simulink model "AFDNFSmodelSPA"  (Simulink 9.0)
settings: Solver=ode45  StartTime=0.0  StopTime=100  FixedStep=1e-3  RelTol=1e-6  EnableMultiTasking=on
InitFcn:
  | run('Methods/AFDSimInit')
values from neighbouring files (symbols this model uses):
  nfs = TransferFunction('Plot','true')    [Main.m]    (also in NFSDatabase.sldd = SI
                Imperial
                28184.4409185639)
undefined symbols (not defined in the file or in its folder): desired, F, K_lat, K_long, Kobsvlat, Kobsvlong, lat, latsys, Light, long, longsys, MIL, Newton, Raphson, sigbuilder_block
libraries: aerolibwind2 x2, sharedutil x1
(part 2 of 3)

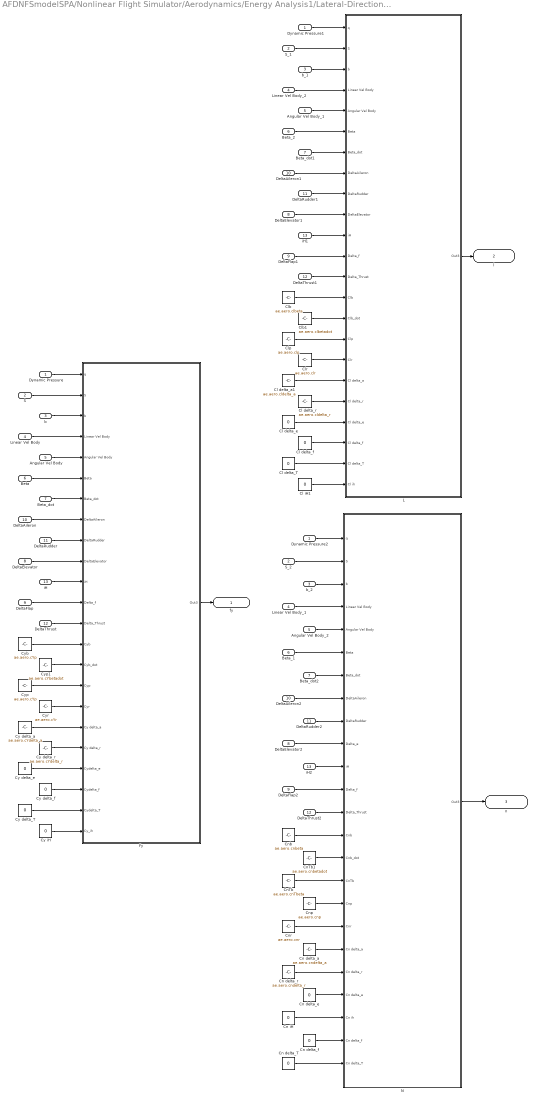
== system AFDNFSmodelSPA/Nonlinear Flight Simulator/Aerodynamics/Energy Analysis1/Lateral-Directional1 ==
  Dynamic Pressure : Inport
  S : Inport  Port=2
  b : Inport  Port=3
  Linear Vel Body : Inport  Port=4
  Angular Vel Body : Inport  Port=5
  Beta : Inport  Port=6
  Beta_dot : Inport  Port=7
  DeltaElevator : Inport  Port=8
  DeltaFlap : Inport  Port=9
  DeltaAileron : Inport  Port=10
  DeltaRudder : Inport  Port=11
  DeltaThrust : Inport  Port=12
  iH : Inport  Port=13
  Angular Vel Body_1 : InportShadow  Port=5
  Angular Vel Body_2 : InportShadow  Port=5
  Beta_1 : InportShadow  Port=6
  Beta_2 : InportShadow  Port=6
  Beta_dot1 : InportShadow  Port=7
  Beta_dot2 : InportShadow  Port=7
  Cl delta_T : Constant  Value=0
  Cl delta_a1 : Constant  Value=ae.aero.cldelta_a
  Cl delta_e : Constant  Value=0
  Cl delta_f : Constant  Value=0
  Cl delta_r : Constant  Value=ae.aero.cldelta_r
  Cl iH1 : Constant  Value=0
  Clb : Constant  Value=ae.aero.clbeta
  Clb1 : Constant  Value=ae.aero.clbetadot
  Clp : Constant  Value=ae.aero.clp
  Clr : Constant  Value=ae.aero.clr
  Cn delta_T : Constant  Value=0
  Cn delta_a : Constant  Value=ae.aero.cndelta_a
  Cn delta_e : Constant  Value=0
  Cn delta_f : Constant  Value=0
  Cn delta_r : Constant  Value=ae.aero.cndelta_r
  Cn iH : Constant  Value=0
  CnTb : Constant  Value=ae.aero.cnTbeta
  CnTb1 : Constant  Value=ae.aero.cnbetadot
  Cnb : Constant  Value=ae.aero.cnbeta
  Cnp : Constant  Value=ae.aero.cnp
  Cnr : Constant  Value=ae.aero.cnr
  Cy delta_T : Constant  Value=0
  Cy delta_a : Constant  Value=ae.aero.cYdelta_a
  Cy delta_e : Constant  Value=0
  Cy delta_f : Constant  Value=0
  Cy delta_r : Constant  Value=ae.aero.cYdelta_r
  Cy iH : Constant  Value=0
  Cyb : Constant  Value=ae.aero.cYp
  Cyp : Constant  Value=ae.aero.cYp
  Cyp1 : Constant  Value=ae.aero.cYbetadot
  Cyr : Constant  Value=ae.aero.cYr
  DeltaAileron1 : InportShadow  Port=10
  DeltaAileron2 : InportShadow  Port=10
  DeltaElevator1 : InportShadow  Port=8
  DeltaElevator2 : InportShadow  Port=8
  DeltaFlap1 : InportShadow  Port=9
  DeltaFlap2 : InportShadow  Port=9
  DeltaRudder1 : InportShadow  Port=11
  DeltaRudder2 : InportShadow  Port=11
  DeltaThrust1 : InportShadow  Port=12
  DeltaThrust2 : InportShadow  Port=12
  Dynamic Pressure1 : InportShadow
  Dynamic Pressure2 : InportShadow
  Fy : Subsystem
  L : Subsystem
  Linear Vel Body_1 : InportShadow  Port=4
  Linear Vel Body_2 : InportShadow  Port=4
  N : Subsystem
  S_1 : InportShadow  Port=2
  S_2 : InportShadow  Port=2
  b_1 : InportShadow  Port=3
  b_2 : InportShadow  Port=3
  iH1 : InportShadow  Port=13
  iH2 : InportShadow  Port=13
  fy : Outport
  l : Outport  Port=2
  n : Outport  Port=3
  wires:
  L/1(Out3) -> l/1
  N/1(Out3) -> n/1
  Fy/1(Out3) -> fy/1
  Dynamic Pressure/1 -> Fy/1(q)
  S/1 -> Fy/2(S)
  b/1 -> Fy/3(b)
  Linear Vel Body/1 -> Fy/4(Linear Vel Body)
  Angular Vel Body/1 -> Fy/5(Angular Vel Body)
  Beta/1 -> Fy/6(Beta)
  Beta_dot/1 -> Fy/7(Beta_dot)
  DeltaAileron/1 -> Fy/8(DeltaAileron)
  DeltaRudder/1 -> Fy/9(DeltaRudder)
  iH/1 -> Fy/11(iH)
  DeltaElevator/1 -> Fy/10(DeltaElevator)
  DeltaFlap/1 -> Fy/12(Delta_f)
  DeltaThrust/1 -> Fy/13(Delta_Thrust)
  DeltaRudder2/1 -> N/9(DeltaRudder)
  DeltaAileron2/1 -> N/8(DeltaAileron)
  Dynamic Pressure2/1 -> N/1(q)
  DeltaThrust2/1 -> N/13(Delta_Thrust)
  b_2/1 -> N/3(b)
  Angular Vel Body_2/1 -> N/5(Angular Vel Body)
  Linear Vel Body_1/1 -> N/4(Linear Vel Body)
  iH2/1 -> N/11(iH)
  Beta_dot2/1 -> N/7(Beta_dot)
  S_2/1 -> N/2(S)
  DeltaElevator2/1 -> N/10(Delta_e)
  DeltaFlap2/1 -> N/12(Delta_f)
  Beta_1/1 -> N/6(Beta)
  Cyb/1 -> Fy/14(Cyb)
  Cyp/1 -> Fy/16(Cyp)
  Cyr/1 -> Fy/17(Cyr)
  Cy delta_a/1 -> Fy/18(Cy delta_a)
  Cy delta_r/1 -> Fy/19(Cy delta_r)
  Cy delta_e/1 -> Fy/20(Cydelta_e)
  Cy delta_f/1 -> Fy/21(Cydelta_f)
  Cy delta_T/1 -> Fy/22(Cydelta_T)
  Cy iH/1 -> Fy/23(Cy_ih)
  Cnb/1 -> N/14(Cnb)
  Cnp/1 -> N/17(Cnp)
  Cn delta_T/1 -> N/24(Cn delta_T)
  CnTb/1 -> N/16(CnTb)
  Cn delta_a/1 -> N/19(Cn delta_a)
  Cn delta_e/1 -> N/21(Cn delta_e)
  Cn delta_r/1 -> N/20(Cn delta_r)
  Cn iH/1 -> N/22(Cn ih)
  Cn delta_f/1 -> N/23(Cn delta_f)
  Cnr/1 -> N/18(Cnr)
  Clb/1 -> L/14(Clb)
  Clp/1 -> L/16(Clp)
  Cl delta_a1/1 -> L/18(Cl delta_a)
  b_1/1 -> L/3(b)
  Dynamic Pressure1/1 -> L/1(q)
  Angular Vel Body_1/1 -> L/5(Angular Vel Body)
  iH1/1 -> L/11(iH)
  DeltaRudder1/1 -> L/9(DeltaRudder)
  DeltaThrust1/1 -> L/13(Delta_Thrust)
  Beta_dot1/1 -> L/7(Beta_dot)
  Beta_2/1 -> L/6(Beta)
  DeltaAileron1/1 -> L/8(DeltaAileron)
  DeltaFlap1/1 -> L/12(Delta_f)
  DeltaElevator1/1 -> L/10(DeltaElevator)
  Linear Vel Body_2/1 -> L/4(Linear Vel Body)
  S_1/1 -> L/2(S)
  Clr/1 -> L/17(Clr)
  Cl delta_e/1 -> L/20(Cl delta_e)
  Cl delta_T/1 -> L/22(Cl delta_T)
  Cl delta_f/1 -> L/21(Cl delta_f)
  Cl delta_r/1 -> L/19(Cl delta_r)
  Cl iH1/1 -> L/23(Cl ih)
  Clb1/1 -> L/15(Clb_dot)
  CnTb1/1 -> N/15(Cnb_dot)
  Cyp1/1 -> Fy/15(Cyb_dot)

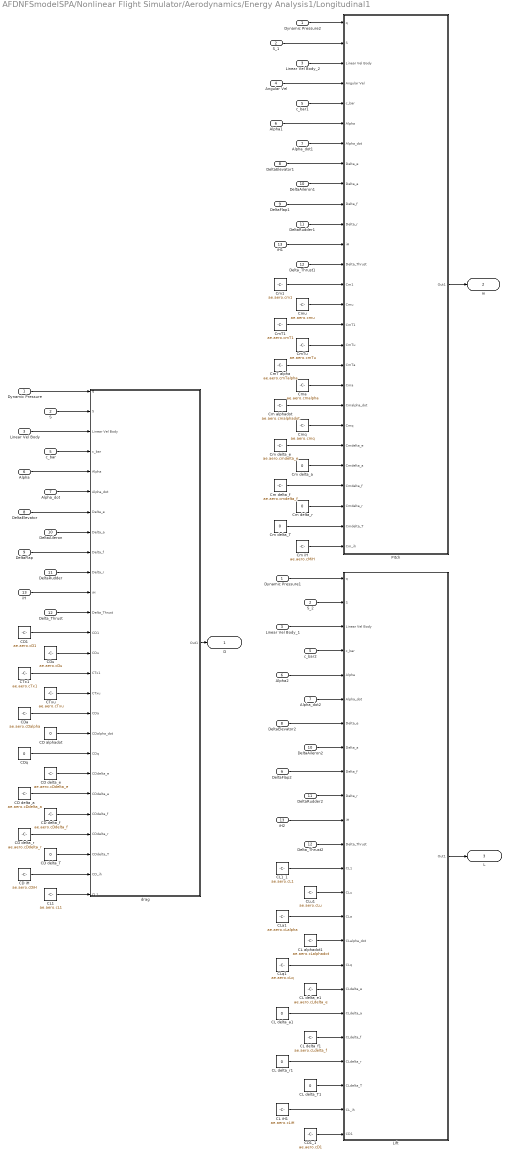
== system AFDNFSmodelSPA/Nonlinear Flight Simulator/Aerodynamics/Energy Analysis1/Longitudinal1 ==
  Dynamic Pressure : Inport
  S : Inport  Port=2
  Linear Vel Body : Inport  Port=3
  Angular Vel : Inport  Port=4
  c_bar : Inport  Port=5
  Alpha : Inport  Port=6
  Alpha_dot : Inport  Port=7
  DeltaElevator : Inport  Port=8
  DeltaFlap : Inport  Port=9
  DeltaAileron : Inport  Port=10
  DeltaRudder : Inport  Port=11
  Delta_Thrust : Inport  Port=12
  iH : Inport  Port=13
  Alpha1 : InportShadow  Port=6
  Alpha2 : InportShadow  Port=6
  Alpha_dot1 : InportShadow  Port=7
  Alpha_dot2 : InportShadow  Port=7
  CD alphadot : Constant  Value=0
  CD delta_T : Constant  Value=0
  CD delta_a : Constant  Value=ae.aero.cDdelta_a
  CD delta_e : Constant  Value=ae.aero.cDdelta_e
  CD delta_f : Constant  Value=ae.aero.cDdelta_f
  CD delta_r : Constant  Value=ae.aero.cDdelta_r
  CD iH : Constant  Value=ae.aero.cDiH
  CD1 : Constant  Value=ae.aero.cD1
  CD1_1 : Constant  Value=ae.aero.cD1
  CDa : Constant  Value=ae.aero.cDalpha
  CDq : Constant  Value=0
  CDu : Constant  Value=ae.aero.cDu
  CL alphadot1 : Constant  Value=ae.aero.cLalphadot
  CL delta_T1 : Constant  Value=0
  CL delta_a1 : Constant  Value=0
  CL delta_e1 : Constant  Value=ae.aero.cLdelta_e
  CL delta_f1 : Constant  Value=ae.aero.cLdelta_f
  CL delta_r1 : Constant  Value=0
  CL iH1 : Constant  Value=ae.aero.cLiH
  CL1 : Constant  Value=ae.aero.cL1
  CL1_1 : Constant  Value=ae.aero.cL1
  CLa1 : Constant  Value=ae.aero.cLalpha
  CLq1 : Constant  Value=ae.aero.cLq
  CLu1 : Constant  Value=ae.aero.cLu
  CTx1 : Constant  Value=ae.aero.cTx1
  CTxu : Constant  Value=ae.aero.cTxu
  Cm alphadot : Constant  Value=ae.aero.cmalphadot
  Cm delta_T : Constant  Value=0
  Cm delta_a : Constant  Value=0
  Cm delta_e : Constant  Value=ae.aero.cmdelta_e
  Cm delta_f : Constant  Value=ae.aero.cmdelta_f
  Cm delta_r : Constant  Value=0
  Cm iH : Constant  Value=ae.aero.cMiH
  Cm1 : Constant  Value=ae.aero.cm1
  CmT alpha : Constant  Value=ae.aero.cmTalpha
  CmT1 : Constant  Value=ae.aero.cmT1
  CmTu : Constant  Value=ae.aero.cmTu
  Cma : Constant  Value=ae.aero.cmalpha
  Cmq : Constant  Value=ae.aero.cmq
  Cmu : Constant  Value=ae.aero.cmu
  DeltaAileron1 : InportShadow  Port=10
  DeltaAileron2 : InportShadow  Port=10
  DeltaElevator1 : InportShadow  Port=8
  DeltaElevator2 : InportShadow  Port=8
  DeltaFlap1 : InportShadow  Port=9
  DeltaFlap2 : InportShadow  Port=9
  DeltaRudder1 : InportShadow  Port=11
  DeltaRudder2 : InportShadow  Port=11
  Delta_Thrust1 : InportShadow  Port=12
  Delta_Thrust2 : InportShadow  Port=12
  Dynamic Pressure1 : InportShadow
  Dynamic Pressure2 : InportShadow
  Lift : Subsystem
  Linear Vel Body_1 : InportShadow  Port=3
  Linear Vel Body_2 : InportShadow  Port=3
  Pitch : Subsystem
  S_1 : InportShadow  Port=2
  S_2 : InportShadow  Port=2
  c_bar1 : InportShadow  Port=5
  c_bar2 : InportShadow  Port=5
  drag : Subsystem
  iH1 : InportShadow  Port=13
  iH2 : InportShadow  Port=13
  D : Outport
  m : Outport  Port=2
  L : Outport  Port=3
  wires:
  DeltaRudder/1 -> drag/10(Delta_r)
  DeltaAileron/1 -> drag/8(Delta_a)
  CDa/1 -> drag/17(CDa)
  Alpha/1 -> drag/5(Alpha)
  CDu/1 -> drag/14(CDu)
  Alpha_dot/1 -> drag/6(Alpha_dot)
  drag/1(Out1) -> D/1
  Lift/1(Out1) -> L/1
  S/1 -> drag/2(S)
  Dynamic Pressure/1 -> drag/1(q)
  Linear Vel Body/1 -> drag/3(Linear Vel Body)
  Delta_Thrust/1 -> drag/12(Delta_Thrust)
  iH/1 -> drag/11(iH)
  CD delta_T/1 -> drag/24(CDdelta_T)
  DeltaElevator/1 -> drag/7(Delta_e)
  DeltaFlap/1 -> drag/9(Delta_f)
  Pitch/1(Out1) -> m/1
  c_bar/1 -> drag/4(c_bar)
  CD alphadot/1 -> drag/18(CDalpha_dot)
  CDq/1 -> drag/19(CDq)
  CD delta_e/1 -> drag/20(CDdelta_e)
  CD delta_a/1 -> drag/21(CDdelta_a)
  CD delta_f/1 -> drag/22(CDdelta_f)
  CD delta_r/1 -> drag/23(CDdelta_r)
  CD iH/1 -> drag/25(CD_ih)
  CTx1/1 -> drag/15(CTx1)
  CD1/1 -> drag/13(CD1)
  CTxu/1 -> drag/16(CTxu)
  DeltaRudder1/1 -> Pitch/11(Delta_r)
  DeltaAileron1/1 -> Pitch/9(Delta_a)
  Alpha1/1 -> Pitch/6(Alpha)
  Alpha_dot1/1 -> Pitch/7(Alpha_dot)
  S_1/1 -> Pitch/2(S)
  Dynamic Pressure2/1 -> Pitch/1(q)
  Linear Vel Body_2/1 -> Pitch/3(Linear Vel Body)
  Delta_Thrust1/1 -> Pitch/13(Delta_Thrust)
  iH1/1 -> Pitch/12(iH)
  DeltaElevator1/1 -> Pitch/8(Delta_e)
  DeltaFlap1/1 -> Pitch/10(Delta_f)
  S_2/1 -> Lift/2(S)
  Dynamic Pressure1/1 -> Lift/1(q)
  Linear Vel Body_1/1 -> Lift/3(Linear Vel Body)
  Delta_Thrust2/1 -> Lift/12(Delta_Thrust)
  c_bar2/1 -> Lift/4(c_bar)
  CL1/1 -> drag/26(CL1)
  iH2/1 -> Lift/11(iH)
  DeltaRudder2/1 -> Lift/10(Delta_r)
  DeltaFlap2/1 -> Lift/9(Delta_f)
  DeltaAileron2/1 -> Lift/8(Delta_a)
  DeltaElevator2/1 -> Lift/7(Delta_e)
  Alpha_dot2/1 -> Lift/6(Alpha_dot)
  Alpha2/1 -> Lift/5(Alpha)
  Angular Vel/1 -> Pitch/4(Angular Vel)
  c_bar1/1 -> Pitch/5(c_bar)
  CD1_1/1 -> Lift/24(CD1)
  CLa1/1 -> Lift/15(CLa)
  CLq1/1 -> Lift/17(CLq)
  CL delta_a1/1 -> Lift/19(CLdelta_a)
  CL delta_r1/1 -> Lift/21(CLdelta_r)
  CL iH1/1 -> Lift/23(CL_ih)
  CL delta_T1/1 -> Lift/22(CLdelta_T)
  CLu1/1 -> Lift/14(CLu)
  CL alphadot1/1 -> Lift/16(CLalpha_dot)
  CL delta_f1/1 -> Lift/20(CLdelta_f)
  CL delta_e1/1 -> Lift/18(CLdelta_e)
  CL1_1/1 -> Lift/13(CL1)
  CmT alpha/1 -> Pitch/18(CmTa)
  Cm alphadot/1 -> Pitch/20(Cmalpha_dot)
  Cm delta_e/1 -> Pitch/22(Cmdelta_e)
  Cm delta_f/1 -> Pitch/24(Cmdelta_f)
  Cm delta_T/1 -> Pitch/26(Cmdelta_T)
  CmT1/1 -> Pitch/16(CmT1)
  Cm1/1 -> Pitch/14(Cm1)
  CmTu/1 -> Pitch/17(CmTu)
  Cmq/1 -> Pitch/21(Cmq)
  Cm delta_a/1 -> Pitch/23(Cmdelta_a)
  Cm delta_r/1 -> Pitch/25(Cmdelta_r)
  Cmu/1 -> Pitch/15(Cmu)
  Cma/1 -> Pitch/19(Cma)
  Cm iH/1 -> Pitch/27(Cm_ih)

== system AFDNFSmodelSPA/Nonlinear Flight Simulator/Aerodynamics/Forces/Aerodynamic  Force ==
  CL : Inport  PortDimensions=1
  CD : Inport  Port=2  PortDimensions=1
  CY : Inport  Port=3  PortDimensions=1
  Dynamic Pressure : Inport  Port=4  PortDimensions=1
  Alpha : Inport  Port=5  PortDimensions=1
  Beta : Inport  Port=6  PortDimensions=1
  ChSign : Gain  Gain=-1  SaturateOnIntegerOverflow=on  OutDataTypeStr=Inherit: Same as input  ParamDataTypeStr=Inherit: Same as input
  ChSign1 : Gain  Gain=-1  SaturateOnIntegerOverflow=on  OutDataTypeStr=Inherit: Same as input  ParamDataTypeStr=Inherit: Same as input
  Mux : Mux  Inputs=3
  Product{,2..4} (4 alike) : Product  SaturateOnIntegerOverflow=on  InputSameDT=on  OutDataTypeStr=Inherit: Same as first input
  Product1 : Product  Multiplication=Matrix(*)  SaturateOnIntegerOverflow=on  InputSameDT=on  OutDataTypeStr=Inherit: Same as first input
  Wind2Body TM : Subsystem
  Wing Area : Constant  Value=nfs.refarea
  Aerodynamic Force : Outport  PortDimensions=[3,1]
  wires:
  Wind2Body TM/1(T_BW) -> Product1/1
  Product1/1 -> Aerodynamic Force/1
  Beta/1 -> Wind2Body TM/2(Beta)
  CD/1 -> ChSign/1
  CL/1 -> ChSign1/1
  Alpha/1 -> Wind2Body TM/1(Alpha)
  Dynamic Pressure/1 -> Product/1
  Wing Area/1 -> Product/2
  Product/1 -> Product2/1, Product3/1, Product4/1
  ChSign/1 -> Product2/2
  CY/1 -> Product3/2
  ChSign1/1 -> Product4/2
  Product2/1 -> Mux/1
  Product3/1 -> Mux/2
  Product4/1 -> Mux/3
  Mux/1 -> Product1/2

== system AFDNFSmodelSPA/Nonlinear Flight Simulator/Aerodynamics/Forces/Drag Coefficient ==
  CL : Inport  PortDimensions=1
  alpha : Inport  Port=2  PortDimensions=1
  DeltaElevator : Inport  Port=3  PortDimensions=1
  DeltaFlap : Inport  Port=4  PortDimensions=1
  DeltaAileron : Inport  Port=5  PortDimensions=1
  DeltaRudder : Inport  Port=6  PortDimensions=1
  Mach : Inport  Port=7  PortDimensions=1
  Abs{,1..4} (5 alike) : Abs  SaturateOnIntegerOverflow=on
  CD0 : Constant  Value=cD0
  CL^2 : Math  Operator=square  SaturateOnIntegerOverflow=on
  Induced Drag : Gain  Gain=nfs.aero.k  SaturateOnIntegerOverflow=on  OutDataTypeStr=Inherit: Same as input  ParamDataTypeStr=Inherit: Same as input
  Sum2 : Sum  Inputs=++++++++  SaturateOnIntegerOverflow=on  InputSameDT=on  OutDataTypeStr=Inherit: Same as first input
  cDM : Gain  Gain=nfs.aero.cDM  SaturateOnIntegerOverflow=on  OutDataTypeStr=Inherit: Same as input  ParamDataTypeStr=Inherit: Same as input
  cDalpha : Gain  Gain=nfs.aero.cDalpha  SaturateOnIntegerOverflow=on  OutDataTypeStr=Inherit: Same as input  ParamDataTypeStr=Inherit: Same as input
  cDdelta_a : Gain  Gain=nfs.aero.cDdelta_a  SaturateOnIntegerOverflow=on  OutDataTypeStr=Inherit: Same as input  ParamDataTypeStr=Inherit: Same as input
  cDdelta_e : Gain  Gain=nfs.aero.cDdelta_e  SaturateOnIntegerOverflow=on  OutDataTypeStr=Inherit: Same as input  ParamDataTypeStr=Inherit: Same as input
  cDdelta_f : Gain  Gain=nfs.aero.cDdelta_f  SaturateOnIntegerOverflow=on  OutDataTypeStr=Inherit: Same as input  ParamDataTypeStr=Inherit: Same as input
  cDdelta_r : Gain  Gain=nfs.aero.cDdelta_r  SaturateOnIntegerOverflow=on  OutDataTypeStr=Inherit: Same as input  ParamDataTypeStr=Inherit: Same as input
  CD : Outport  PortDimensions=1
  wires:
  Sum2/1 -> CD/1
  DeltaRudder/1 -> cDdelta_r/1
  DeltaAileron/1 -> cDdelta_a/1
  DeltaElevator/1 -> cDdelta_e/1
  DeltaFlap/1 -> cDdelta_f/1
  Mach/1 -> cDM/1
  CL/1 -> CL^2/1
  cDdelta_r/1 -> Abs3/1
  cDdelta_a/1 -> Abs2/1
  cDdelta_e/1 -> Abs1/1
  cDdelta_f/1 -> Abs/1
  Induced Drag/1 -> Sum2/2
  CD0/1 -> Sum2/1
  CL^2/1 -> Induced Drag/1
  alpha/1 -> cDalpha/1
  cDalpha/1 -> Abs4/1
  Abs/1 -> Sum2/4
  Abs1/1 -> Sum2/5
  Abs2/1 -> Sum2/6
  Abs3/1 -> Sum2/7
  cDM/1 -> Sum2/8
  Abs4/1 -> Sum2/3

== system AFDNFSmodelSPA/Nonlinear Flight Simulator/Aerodynamics/Forces/Lift Coefficient ==
  Linear Velocity : Inport  PortDimensions=[3 1]
  Alpha : Inport  Port=2  PortDimensions=1
  DeltaElevator : Inport  Port=3  PortDimensions=1
  DeltaFlap : Inport  Port=4  PortDimensions=1
  Alphadot : Inport  Port=5  PortDimensions=1
  Q : Inport  Port=6  PortDimensions=1
  Mach : Inport  Port=7  PortDimensions=1
  1 : Gain  Gain=2  SaturateOnIntegerOverflow=on  OutDataTypeStr=Inherit: Same as input  ParamDataTypeStr=Inherit: Same as input
  CL*c/(2V) : Product  Inputs=**/  SaturateOnIntegerOverflow=on  InputSameDT=on  OutDataTypeStr=Inherit: Same as first input
  CL0 : Constant  Value=cL0
  CLM : Gain  Gain=nfs.aero.cLM  SaturateOnIntegerOverflow=on  OutDataTypeStr=Inherit: Same as input  ParamDataTypeStr=Inherit: Same as input
  Sum1 : Sum  SaturateOnIntegerOverflow=on  InputSameDT=on  OutDataTypeStr=Inherit: Same as first input
  Sum3 : Sum  Inputs=++++++  SaturateOnIntegerOverflow=on  InputSameDT=on  OutDataTypeStr=Inherit: Same as first input
  Velocity Magnitude : Subsystem
  Wing chord1 : Constant  Value=meanchord
  cLalpha : Gain  Gain=nfs.aero.cLalpha  SaturateOnIntegerOverflow=on  OutDataTypeStr=Inherit: Same as input  ParamDataTypeStr=Inherit: Same as input
  cLalphadot : Gain  Gain=nfs.aero.cLalphadot  SaturateOnIntegerOverflow=on  OutDataTypeStr=Inherit: Same as input  ParamDataTypeStr=Inherit: Same as input
  cLdelta_e : Gain  Gain=nfs.aero.cLdelta_e  SaturateOnIntegerOverflow=on  OutDataTypeStr=Inherit: Same as input  ParamDataTypeStr=Inherit: Same as input
  cLdelta_f : Gain  Gain=nfs.aero.cLdelta_f  SaturateOnIntegerOverflow=on  OutDataTypeStr=Inherit: Same as input  ParamDataTypeStr=Inherit: Same as input
  cLq : Gain  Gain=nfs.aero.cLq  SaturateOnIntegerOverflow=on  OutDataTypeStr=Inherit: Same as input  ParamDataTypeStr=Inherit: Same as input
  CL : Outport  PortDimensions=1
  wires:
  Sum3/1 -> CL/1
  Q/1 -> cLq/1
  Alphadot/1 -> cLalphadot/1
  Velocity Magnitude/1(Velocity Magnitude) -> 1/1
  Linear Velocity/1 -> Velocity Magnitude/1(Velocity)
  Mach/1 -> CLM/1
  CL*c/(2V)/1 -> Sum3/5
  cLdelta_f/1 -> Sum3/4
  cLdelta_e/1 -> Sum3/3
  cLalpha/1 -> Sum3/2
  CL0/1 -> Sum3/1
  Sum1/1 -> CL*c/(2V)/1
  cLalphadot/1 -> Sum1/1
  DeltaFlap/1 -> cLdelta_f/1
  DeltaElevator/1 -> cLdelta_e/1
  Alpha/1 -> cLalpha/1
  cLq/1 -> Sum1/2
  Wing chord1/1 -> CL*c/(2V)/2
  1/1 -> CL*c/(2V)/3
  CLM/1 -> Sum3/6

== system AFDNFSmodelSPA/Nonlinear Flight Simulator/Aerodynamics/Forces/SideForce Coefficient ==
  Linear Velocity : Inport  PortDimensions=[3 1]
  Beta : Inport  Port=2  PortDimensions=1
  P : Inport  Port=3  PortDimensions=1
  R : Inport  Port=4  PortDimensions=1
  DeltaAileron : Inport  Port=5  PortDimensions=1
  DeltaRudder : Inport  Port=6  PortDimensions=1
  2 : Gain  Gain=2  SaturateOnIntegerOverflow=on  OutDataTypeStr=Inherit: Same as input  ParamDataTypeStr=Inherit: Same as input
  CY*b/(2V) : Product  Inputs=**/  SaturateOnIntegerOverflow=on  InputSameDT=on  OutDataTypeStr=Inherit: Same as first input
  Sum : Sum  SaturateOnIntegerOverflow=on  InputSameDT=on  OutDataTypeStr=Inherit: Same as first input
  Sum2 : Sum  Inputs=++++  SaturateOnIntegerOverflow=on  InputSameDT=on  OutDataTypeStr=Inherit: Same as first input
  Velocity Magnitude : Subsystem
  Wing span : Constant  Value=nfs.span
  cYbeta : Gain  Gain=nfs.aero.cYbeta  SaturateOnIntegerOverflow=on  OutDataTypeStr=Inherit: Same as input  ParamDataTypeStr=Inherit: Same as input
  cYdelta_a : Gain  Gain=nfs.aero.cYdelta_a  SaturateOnIntegerOverflow=on  OutDataTypeStr=Inherit: Same as input  ParamDataTypeStr=Inherit: Same as input
  cYdelta_r : Gain  Gain=nfs.aero.cYdelta_r  SaturateOnIntegerOverflow=on  OutDataTypeStr=Inherit: Same as input  ParamDataTypeStr=Inherit: Same as input
  cYp : Gain  Gain=nfs.aero.cYp  SaturateOnIntegerOverflow=on  OutDataTypeStr=Inherit: Same as input  ParamDataTypeStr=Inherit: Same as input
  cYr : Gain  Gain=nfs.aero.cYr  SaturateOnIntegerOverflow=on  OutDataTypeStr=Inherit: Same as input  ParamDataTypeStr=Inherit: Same as input
  CY : Outport
  wires:
  Sum2/1 -> CY/1
  R/1 -> cYr/1
  P/1 -> cYp/1
  DeltaRudder/1 -> cYdelta_r/1
  DeltaAileron/1 -> cYdelta_a/1
  Velocity Magnitude/1(Velocity Magnitude) -> 2/1
  Linear Velocity/1 -> Velocity Magnitude/1(Velocity)
  Beta/1 -> cYbeta/1
  CY*b/(2V)/1 -> Sum2/4
  cYdelta_r/1 -> Sum2/3
  cYdelta_a/1 -> Sum2/2
  cYbeta/1 -> Sum2/1
  2/1 -> CY*b/(2V)/3
  Wing span/1 -> CY*b/(2V)/2
  Sum/1 -> CY*b/(2V)/1
  cYr/1 -> Sum/2
  cYp/1 -> Sum/1

== system AFDNFSmodelSPA/Nonlinear Flight Simulator/Aerodynamics/Forces/Thrust ==
  Manual Switch : ManualSwitch  CurrentSetting=0
  Mux1 : Mux  Inputs=3
  Product : Product  RndMeth=Zero
  Signal Builder : Subsystem  Tag=STV Subsys  LoadFcn=sigbuilder_block('load');  StartFcn=sigbuilder_block('start');  StopFcn=sigbuilder_block('stop');  ClipboardFcn=sigbuilder_block('clipboard');  mask(Sigbuilder block){tuvar=[0:10]}
      mask help: Simulink:masks:SigbuilderBlock_MD
      mask init:
      | if ~strcmp(get_param(bdroot(gcbh),'SimulationStatus'),'stopped') tuvar = sigbuilder_block('maskInit'); end
      settings: CopyFcn=sigbuilder_block('copy');  DeleteFcn=sigbuilder_block('delete');  ModelCloseFcn=sigbuilder_block('modelClose');  PreSaveFcn=sigbuilder_block('preSave');  PauseFcn=sigbuilder_block('pause');  ContinueFcn=sigbuilder_block('continue');  NameChangeFcn=sigbuilder_block('namechange');  OpenFcn=sigbuilder_block('open',[437.25 199.5 550.5 399.75 ]);  CloseFcn=sigbuilder_block('close');
      mask Display: plot(0, 0, 100, 100,[2, 2, 32, 32, 2], [68, 8, 8, 68, 68],[32, 2], [38, 38], [32, 19, 2],[53, 60, 44], [32, 17, 17, 2],[16, 16, 31, 31]);txt = getActiveGroup(gcbh);text(2, 100, txt,'verticalAlignment', 'top');
  Throttle : Gain
  Trim Thrust1 : Constant  Value=nfs.trim.thrust*cos(nfs.tmisalign)
  Trim Thrust2 : Constant  Value=nfs.trim.thrust*sin(nfs.tmisalign)
  Trim Thrust3 : Constant  Value=0
  Trim Thrust4 : Constant
  Thrust : Outport  PortDimensions=[3,1]
  wires:
  Mux1/1 -> Throttle/1
  Trim Thrust3/1 -> Mux1/3
  Trim Thrust2/1 -> Mux1/2
  Trim Thrust1/1 -> Mux1/1
  Throttle/1 -> Product/1
  Product/1 -> Thrust/1
  Manual Switch/1 -> Product/2
  Signal Builder/1(ThrustDeviation) -> Manual Switch/1
  Trim Thrust4/1 -> Manual Switch/2

== system AFDNFSmodelSPA/Nonlinear Flight Simulator/Aerodynamics/Forces/Weight ==
  note: theta
  note: phi
  Attitute : Inport  PortDimensions=[3,1]
  Demux : Demux  Outputs=3
  Gain1 : Gain  Gain=-1
  Mux1 : Mux  Inputs=3
  Product{2..6} (5 alike) : Product  RndMeth=Zero
  Terminator4 : Terminator
  Trigonometric Function1 : Trigonometry  Operator=cos
  Trigonometric Function2 : Trigonometry
  Trigonometric Function3 : Trigonometry  Operator=cos
  Trigonometric Function4 : Trigonometry
  Weight Force : Constant  Value=nfs.weight
  Weight : Outport  PortDimensions=[3,1]
  wires:
  Mux1/1 -> Weight/1
  Product6/1 -> Mux1/3
  Product3/1 -> Mux1/2
  Product2/1 -> Mux1/1
  Product5/1 -> Product6/2
  Product4/1 -> Product3/1
  Trigonometric Function1/1 -> Product5/2
  Trigonometric Function4/1 -> Product4/1
  Trigonometric Function3/1 -> Product5/1, Product4/2
  Trigonometric Function2/1 -> Gain1/1
  Weight Force/1 -> Product6/1, Product3/2, Product2/2
  Gain1/1 -> Product2/1
  Demux/3 -> Terminator4/1
  Attitute/1 -> Demux/1
  Demux/2 -> Trigonometric Function3/1, Trigonometric Function2/1
  Demux/1 -> Trigonometric Function1/1, Trigonometric Function4/1

== system AFDNFSmodelSPA/Nonlinear Flight Simulator/Aerodynamics/Moments/Aerodynamic Moment  ==
  Cl : Inport
  Cm : Inport  Port=2
  Cn : Inport  Port=3
  Dynamic Pressure : Inport  Port=4
  Alpha : Inport  Port=5  PortDimensions=1
  Beta : Inport  Port=6  PortDimensions=1
  Dynamic Pressure1 : InportShadow  Port=4
  Dynamic Pressure2 : InportShadow  Port=4
  Mux : Mux  Inputs=3
  Pitch : Product  Inputs=4  SaturateOnIntegerOverflow=on  InputSameDT=on  OutDataTypeStr=Inherit: Same as first input
  Product1 : Product  Commented=on  Multiplication=Matrix(*)  SaturateOnIntegerOverflow=on  InputSameDT=on  OutDataTypeStr=Inherit: Same as first input
  Roll : Product  Inputs=4  SaturateOnIntegerOverflow=on  InputSameDT=on  OutDataTypeStr=Inherit: Same as first input
  Wind2Body TM : Subsystem  Commented=on
  Wing area : Constant  Value=nfs.refarea
  Wing chord : Constant  Value=nfs.meanchord
  Wing span : Constant  Value=nfs.span
  Wing span2 : Constant  Value=nfs.span
  Yaw : Product  Inputs=4  SaturateOnIntegerOverflow=on  InputSameDT=on  OutDataTypeStr=Inherit: Same as first input
  Aerodynamic Moment : Outport  PortDimensions=[3,1]
  wires:
  Yaw/1 -> Mux/3
  Pitch/1 -> Mux/2
  Roll/1 -> Mux/1
  Wing area/1 -> Yaw/2, Roll/2, Pitch/2
  Wing span2/1 -> Yaw/3
  Dynamic Pressure2/1 -> Yaw/1
  Dynamic Pressure1/1 -> Pitch/1
  Cl/1 -> Roll/4
  Cm/1 -> Pitch/4
  Cn/1 -> Yaw/4
  Dynamic Pressure/1 -> Roll/1
  Wing chord/1 -> Pitch/3
  Wing span/1 -> Roll/3
  Wind2Body TM/1(T_BW) -> Product1/1
  Beta/1 -> Wind2Body TM/2(Beta)
  Alpha/1 -> Wind2Body TM/1(Alpha)
  Mux/1 -> Aerodynamic Moment/1

== system AFDNFSmodelSPA/Nonlinear Flight Simulator/Aerodynamics/Moments/Pitch Moment Coefficient ==
  Linear Velocity : Inport
  Alpha : Inport  Port=2
  Q : Inport  Port=3
  DeltaElevator : Inport  Port=4
  DeltaFlap : Inport  Port=5
  Alphadot : Inport  Port=6  PortDimensions=1
  Mach : Inport  Port=7  PortDimensions=1
  2 : Gain  Gain=2  SaturateOnIntegerOverflow=on  OutDataTypeStr=Inherit: Same as input  ParamDataTypeStr=Inherit: Same as input
  Cm*c/(2V) : Product  Inputs=**/  SaturateOnIntegerOverflow=on  InputSameDT=on  OutDataTypeStr=Inherit: Same as first input
  Cm0 : Constant  Value=nfs.aero.cm0
  Scope{1..7} (7 alike) : Scope
  Sum : Sum  SaturateOnIntegerOverflow=on  InputSameDT=on  OutDataTypeStr=Inherit: Same as first input
  Sum2 : Sum  Inputs=++++++  SaturateOnIntegerOverflow=on  InputSameDT=on  OutDataTypeStr=Inherit: Same as first input
  Velocity Magnitude : Subsystem
  Wing chord : Constant  Value=nfs.meanchord
  cmM : Gain  Gain=nfs.aero.cmM  SaturateOnIntegerOverflow=on  OutDataTypeStr=Inherit: Same as input  ParamDataTypeStr=Inherit: Same as input
  cmalpha : Gain  Gain=nfs.aero.cmalpha  SaturateOnIntegerOverflow=on  OutDataTypeStr=Inherit: Same as input  ParamDataTypeStr=Inherit: Same as input
  cmalphadot : Gain  Gain=nfs.aero.cmalphadot  SaturateOnIntegerOverflow=on  OutDataTypeStr=Inherit: Same as input  ParamDataTypeStr=Inherit: Same as input
  cmdelta_e : Gain  Gain=nfs.aero.cmdelta_e  SaturateOnIntegerOverflow=on  OutDataTypeStr=Inherit: Same as input  ParamDataTypeStr=Inherit: Same as input
  cmdelta_f : Gain  Gain=nfs.aero.cmdelta_f  SaturateOnIntegerOverflow=on  OutDataTypeStr=Inherit: Same as input  ParamDataTypeStr=Inherit: Same as input
  cmq : Gain  Gain=nfs.aero.cmq  SaturateOnIntegerOverflow=on  OutDataTypeStr=Inherit: Same as input  ParamDataTypeStr=Inherit: Same as input
  Cm : Outport  PortDimensions=1
  wires:
  Sum2/1 -> Cm/1
  Mach/1 -> cmM/1
  Q/1 -> cmq/1
  Alphadot/1 -> cmalphadot/1
  DeltaElevator/1 -> cmdelta_e/1
  DeltaFlap/1 -> cmdelta_f/1
  Alpha/1 -> cmalpha/1
  Velocity Magnitude/1(Velocity Magnitude) -> 2/1
  Linear Velocity/1 -> Velocity Magnitude/1(Velocity)
  cmM/1 -> Sum2/6, Scope6/1
  Cm*c/(2V)/1 -> Sum2/5
  cmdelta_e/1 -> Sum2/4, Scope3/1
  cmdelta_f/1 -> Sum2/3, Scope2/1
  cmalpha/1 -> Sum2/2, Scope1/1
  Cm0/1 -> Sum2/1, Scope7/1
  Sum/1 -> Cm*c/(2V)/1
  cmalphadot/1 -> Sum/1, Scope4/1
  cmq/1 -> Sum/2, Scope5/1
  Wing chord/1 -> Cm*c/(2V)/2
  2/1 -> Cm*c/(2V)/3

== system AFDNFSmodelSPA/Nonlinear Flight Simulator/Aerodynamics/Moments/Roll Moment Coefficient ==
  Linear Velocity : Inport
  Beta : Inport  Port=2  PortDimensions=1
  P : Inport  Port=3
  R : Inport  Port=4
  DeltaAileron : Inport  Port=5
  DeltaRudder : Inport  Port=6
  2 : Gain  Gain=2  SaturateOnIntegerOverflow=on  OutDataTypeStr=Inherit: Same as input  ParamDataTypeStr=Inherit: Same as input
  Cl*b/(2V) : Product  Inputs=**/  SaturateOnIntegerOverflow=on  InputSameDT=on  OutDataTypeStr=Inherit: Same as first input
  Sum : Sum  SaturateOnIntegerOverflow=on  InputSameDT=on  OutDataTypeStr=Inherit: Same as first input
  Sum2 : Sum  Inputs=++++  SaturateOnIntegerOverflow=on  InputSameDT=on  OutDataTypeStr=Inherit: Same as first input
  Velocity Magnitude : Subsystem
  Wing span : Constant  Value=nfs.span
  clbeta : Gain  Gain=nfs.aero.clbeta  SaturateOnIntegerOverflow=on  OutDataTypeStr=Inherit: Same as input  ParamDataTypeStr=Inherit: Same as input
  cldelta_a : Gain  Gain=nfs.aero.cldelta_a  SaturateOnIntegerOverflow=on  OutDataTypeStr=Inherit: Same as input  ParamDataTypeStr=Inherit: Same as input
  cldelta_r : Gain  Gain=nfs.aero.cldelta_r  SaturateOnIntegerOverflow=on  OutDataTypeStr=Inherit: Same as input  ParamDataTypeStr=Inherit: Same as input
  clp : Gain  Gain=nfs.aero.clp  SaturateOnIntegerOverflow=on  OutDataTypeStr=Inherit: Same as input  ParamDataTypeStr=Inherit: Same as input
  clr : Gain  Gain=nfs.aero.clr  SaturateOnIntegerOverflow=on  OutDataTypeStr=Inherit: Same as input  ParamDataTypeStr=Inherit: Same as input
  Cl : Outport  PortDimensions=1
  wires:
  Sum2/1 -> Cl/1
  R/1 -> clr/1
  P/1 -> clp/1
  DeltaRudder/1 -> cldelta_r/1
  DeltaAileron/1 -> cldelta_a/1
  Beta/1 -> clbeta/1
  Velocity Magnitude/1(Velocity Magnitude) -> 2/1
  Linear Velocity/1 -> Velocity Magnitude/1(Velocity)
  Cl*b/(2V)/1 -> Sum2/4
  cldelta_r/1 -> Sum2/3
  cldelta_a/1 -> Sum2/2
  clbeta/1 -> Sum2/1
  2/1 -> Cl*b/(2V)/3
  Wing span/1 -> Cl*b/(2V)/2
  Sum/1 -> Cl*b/(2V)/1
  clr/1 -> Sum/2
  clp/1 -> Sum/1

== system AFDNFSmodelSPA/Nonlinear Flight Simulator/Aerodynamics/Moments/Yaw Moment Coefficient ==
  Linear Velocity : Inport
  beta : Inport  Port=2  PortDimensions=1
  P : Inport  Port=3
  R : Inport  Port=4
  DeltaAileron : Inport  Port=5
  DeltaRudder : Inport  Port=6
  2 : Gain  Gain=2  SaturateOnIntegerOverflow=on  OutDataTypeStr=Inherit: Same as input  ParamDataTypeStr=Inherit: Same as input
  Cn*b/(2V) : Product  Inputs=**/  SaturateOnIntegerOverflow=on  InputSameDT=on  OutDataTypeStr=Inherit: Same as first input
  Sum : Sum  SaturateOnIntegerOverflow=on  InputSameDT=on  OutDataTypeStr=Inherit: Same as first input
  Sum2 : Sum  Inputs=++++  SaturateOnIntegerOverflow=on  InputSameDT=on  OutDataTypeStr=Inherit: Same as first input
  Velocity Magnitude : Subsystem
  Wing span : Constant  Value=nfs.span
  cnbeta : Gain  Gain=nfs.aero.cnbeta  SaturateOnIntegerOverflow=on  OutDataTypeStr=Inherit: Same as input  ParamDataTypeStr=Inherit: Same as input
  cndelta_a : Gain  Gain=nfs.aero.cndelta_a  SaturateOnIntegerOverflow=on  OutDataTypeStr=Inherit: Same as input  ParamDataTypeStr=Inherit: Same as input
  cndelta_r : Gain  Gain=nfs.aero.cndelta_r  SaturateOnIntegerOverflow=on  OutDataTypeStr=Inherit: Same as input  ParamDataTypeStr=Inherit: Same as input
  cnp : Gain  Gain=nfs.aero.cnp  SaturateOnIntegerOverflow=on  OutDataTypeStr=Inherit: Same as input  ParamDataTypeStr=Inherit: Same as input
  cnr : Gain  Gain=nfs.aero.cnr  SaturateOnIntegerOverflow=on  OutDataTypeStr=Inherit: Same as input  ParamDataTypeStr=Inherit: Same as input
  Cn : Outport  PortDimensions=1
  wires:
  Sum2/1 -> Cn/1
  R/1 -> cnr/1
  P/1 -> cnp/1
  DeltaRudder/1 -> cndelta_r/1
  DeltaAileron/1 -> cndelta_a/1
  beta/1 -> cnbeta/1
  Velocity Magnitude/1(Velocity Magnitude) -> 2/1
  Linear Velocity/1 -> Velocity Magnitude/1(Velocity)
  cnp/1 -> Sum/1
  cnr/1 -> Sum/2
  Sum/1 -> Cn*b/(2V)/1
  Wing span/1 -> Cn*b/(2V)/2
  2/1 -> Cn*b/(2V)/3
  cnbeta/1 -> Sum2/1
  cndelta_a/1 -> Sum2/2
  cndelta_r/1 -> Sum2/3
  Cn*b/(2V)/1 -> Sum2/4

== system AFDNFSmodelSPA/Nonlinear Flight Simulator/Aerodynamics/Turbulence/Velocity Magnitude ==
  Velocity : Inport
  Dot Product : DotProduct  InputSameDT=on  OutDataTypeStr=Inherit: Inherit via internal rule
  Sqrt : Sqrt  SaturateOnIntegerOverflow=on
  Velocity Magnitude : Outport
  wires:
  Sqrt/1 -> Velocity Magnitude/1  "abs(V)"
  Velocity/1 -> Dot Product/2, Dot Product/1
  Dot Product/1 -> Sqrt/1

== system AFDNFSmodelSPA/Nonlinear Flight Simulator/Aerodynamics/Turbulence/Velocity Magnitude1 ==
  Velocity : Inport
  Dot Product : DotProduct  InputSameDT=on  OutDataTypeStr=Inherit: Inherit via internal rule
  Sqrt : Sqrt  SaturateOnIntegerOverflow=on
  Velocity Magnitude : Outport
  wires:
  Dot Product/1 -> Sqrt/1
  Velocity/1 -> Dot Product/1, Dot Product/2
  Sqrt/1 -> Velocity Magnitude/1  "abs(V)"

== system AFDNFSmodelSPA/OnBoardComputer/Control System/Trim Offset +  Reference Excitation/Doublet Generated Signal ==
  Constant : Constant  Value=[0;0;0]
  Constant2 : Constant  Value=nfs.trim.delta_e
  Doublet : Subsystem  mask{T_start=10, amp=deg2rad(2), span=1, sampletime=0}
      mask prompts: T_start "Doublet Time"; amp "Amplitude"; span "Time Span"; sampletime "Sample Time"
      mask Display: plot([0,1,1,2,2,3,3,4],[0,0,1,1,-1,-1,0,0])
  Mux : Mux  Inputs=2
  Sum : Sum  Inputs=|++
  Doublet Out : Outport
  wires:
  Sum/1 -> Mux/1
  Constant/1 -> Mux/2
  Doublet/1(Out1) -> Sum/1
  Constant2/1 -> Sum/2
  Mux/1 -> Doublet Out/1

== system AFDNFSmodelSPA/OnBoardComputer/Control System/Trim Offset +  Reference Excitation/Triangular signal span 10 sec ==
  Constant1 : Constant  Value=0
  Constant2 : Constant  Value=nfs.trim.delta_e
  Constant3 : Constant  Value=0
  Constant4 : Constant  Value=0
  Gain{,1..3} (4 alike) : Gain  Gain=pi/180
  Gain4 : Gain
  Gain5 : Gain  Gain=0
  Gain6 : Gain  Gain=0
  Gain7 : Gain
  Mux : Mux
  Signal Builder1 : Subsystem  Tag=STV Subsys  LoadFcn=sigbuilder_block('load');  StartFcn=sigbuilder_block('start');  StopFcn=sigbuilder_block('stop');  ClipboardFcn=sigbuilder_block('clipboard');  mask(Sigbuilder block){tuvar=[0:10]}
      mask help: Simulink:masks:SigbuilderBlock_MD
      mask init:
      | if ~strcmp(get_param(bdroot(gcbh),'SimulationStatus'),'stopped') tuvar = sigbuilder_block('maskInit'); end
      settings: CopyFcn=sigbuilder_block('copy');  DeleteFcn=sigbuilder_block('delete');  ModelCloseFcn=sigbuilder_block('modelClose');  PreSaveFcn=sigbuilder_block('preSave');  PauseFcn=sigbuilder_block('pause');  ContinueFcn=sigbuilder_block('continue');  NameChangeFcn=sigbuilder_block('namechange');  OpenFcn=sigbuilder_block('open',[437.4 199.2 550.2 400.2 ]);  CloseFcn=sigbuilder_block('close');
      mask Display: plot(0, 0, 100, 100,[2, 2, 32, 32, 2], [68, 8, 8, 68, 68],[32, 2], [38, 38], [32, 19, 2],[53, 60, 44], [32, 17, 17, 2],[16, 16, 31, 31]);txt = getActiveGroup(gcbh);text(2, 100, txt,'verticalAlignment', 'top');
  Signal Builder2 : Subsystem  Tag=STV Subsys  LoadFcn=sigbuilder_block('load');  StartFcn=sigbuilder_block('start');  StopFcn=sigbuilder_block('stop');  ClipboardFcn=sigbuilder_block('clipboard');  mask(Sigbuilder block){tuvar=[0:10]}
      mask help: Simulink:masks:SigbuilderBlock_MD
      mask init:
      | if ~strcmp(get_param(bdroot(gcbh),'SimulationStatus'),'stopped') tuvar = sigbuilder_block('maskInit'); end
      settings: CopyFcn=sigbuilder_block('copy');  DeleteFcn=sigbuilder_block('delete');  ModelCloseFcn=sigbuilder_block('modelClose');  PreSaveFcn=sigbuilder_block('preSave');  PauseFcn=sigbuilder_block('pause');  ContinueFcn=sigbuilder_block('continue');  NameChangeFcn=sigbuilder_block('namechange');  OpenFcn=sigbuilder_block('open',[437.25 199.5 550.5 399.75 ]);  CloseFcn=sigbuilder_block('close');
      mask Display: plot(0, 0, 100, 100,[2, 2, 32, 32, 2], [68, 8, 8, 68, 68],[32, 2], [38, 38], [32, 19, 2],[53, 60, 44], [32, 17, 17, 2],[16, 16, 31, 31]);txt = getActiveGroup(gcbh);text(2, 100, txt,'verticalAlignment', 'top');
  Signal Builder3 : Subsystem  Tag=STV Subsys  LoadFcn=sigbuilder_block('load');  StartFcn=sigbuilder_block('start');  StopFcn=sigbuilder_block('stop');  ClipboardFcn=sigbuilder_block('clipboard');  mask(Sigbuilder block){tuvar=[0:10]}
      mask help: Simulink:masks:SigbuilderBlock_MD
      mask init:
      | if ~strcmp(get_param(bdroot(gcbh),'SimulationStatus'),'stopped') tuvar = sigbuilder_block('maskInit'); end
      settings: CopyFcn=sigbuilder_block('copy');  DeleteFcn=sigbuilder_block('delete');  ModelCloseFcn=sigbuilder_block('modelClose');  PreSaveFcn=sigbuilder_block('preSave');  PauseFcn=sigbuilder_block('pause');  ContinueFcn=sigbuilder_block('continue');  NameChangeFcn=sigbuilder_block('namechange');  OpenFcn=sigbuilder_block('open',[437.4 199.2 550.2 400.2 ]);  CloseFcn=sigbuilder_block('close');
      mask Display: plot(0, 0, 100, 100,[2, 2, 32, 32, 2], [68, 8, 8, 68, 68],[32, 2], [38, 38], [32, 19, 2],[53, 60, 44], [32, 17, 17, 2],[16, 16, 31, 31]);txt = getActiveGroup(gcbh);text(2, 100, txt,'verticalAlignment', 'top');
  Signal Builder4 : Subsystem  Tag=STV Subsys  LoadFcn=sigbuilder_block('load');  StartFcn=sigbuilder_block('start');  StopFcn=sigbuilder_block('stop');  ClipboardFcn=sigbuilder_block('clipboard');  mask(Sigbuilder block){tuvar=[0:10]}
      mask help: Simulink:masks:SigbuilderBlock_MD
      mask init:
      | if ~strcmp(get_param(bdroot(gcbh),'SimulationStatus'),'stopped') tuvar = sigbuilder_block('maskInit'); end
      settings: CopyFcn=sigbuilder_block('copy');  DeleteFcn=sigbuilder_block('delete');  ModelCloseFcn=sigbuilder_block('modelClose');  PreSaveFcn=sigbuilder_block('preSave');  PauseFcn=sigbuilder_block('pause');  ContinueFcn=sigbuilder_block('continue');  NameChangeFcn=sigbuilder_block('namechange');  OpenFcn=sigbuilder_block('open',[437.4 199.2 550.2 400.2 ]);  CloseFcn=sigbuilder_block('close');
      mask Display: plot(0, 0, 100, 100,[2, 2, 32, 32, 2], [68, 8, 8, 68, 68],[32, 2], [38, 38], [32, 19, 2],[53, 60, 44], [32, 17, 17, 2],[16, 16, 31, 31]);txt = getActiveGroup(gcbh);text(2, 100, txt,'verticalAlignment', 'top');
  Sum{,1..3} (4 alike) : Sum  Inputs=++|
  Tri : Outport
  wires:
  Mux/1 -> Tri/1
  Signal Builder1/1(Normalized Elevator(deg)) -> Gain/1
  Constant2/1 -> Sum/1
  Gain/1 -> Sum/2
  Signal Builder2/1(Normalized Flap(deg)) -> Gain1/1
  Constant1/1 -> Sum1/1
  Gain1/1 -> Sum1/2
  Signal Builder3/1(Normalized Alileron(deg)) -> Gain2/1
  Constant3/1 -> Sum2/1
  Gain2/1 -> Sum2/2
  Signal Builder4/1(Normalized Rudder(deg)) -> Gain3/1
  Constant4/1 -> Sum3/1
  Gain3/1 -> Sum3/2
  Sum/1 -> Gain7/1
  Sum1/1 -> Gain6/1
  Sum2/1 -> Gain5/1
  Sum3/1 -> Gain4/1
  Gain4/1 -> Mux/4
  Gain5/1 -> Mux/3
  Gain6/1 -> Mux/2
  Gain7/1 -> Mux/1

== system AFDNFSmodelSPA/OnBoardComputer/Control System/Unfinished Controllers (State-Feedback)/Full-State Feedback Servo ==
  States : Inport
  Gain : Gain  Gain=-K_long  Multiplication=Matrix(K*u) (u vector)
  Gain1 : Gain  Gain=-K_lat  Multiplication=Matrix(K*u) (u vector)
  Selector1 : Selector  InputPortWidth=9  IndexOptions=Index vector (dialog)  Indices=[5:9]  OutputSizes=1
  Selector3 : Selector  InputPortWidth=9  IndexOptions=Index vector (dialog)  Indices=[1:4]  OutputSizes=1
  Longitudinal Control : Outport
  Lateral-Directional Control : Outport  Port=2
  wires:
  Gain1/1 -> Lateral-Directional Control/1
  Gain/1 -> Longitudinal Control/1
  Selector1/1 -> Gain1/1  "Lateral-Directional"
  Selector3/1 -> Gain/1  "Longitudinal"
  States/1 -> Selector1/1, Selector3/1

== system AFDNFSmodelSPA/OnBoardComputer/Control System/Unfinished Controllers (State-Feedback)/Full-State Observer Servo ==
  States : Inport  PortDimensions=[9,1]
  U : Inport  Port=2  PortDimensions=[4,1]
  A : Gain  Gain=longsys.a  Multiplication=Matrix(K*u)
  A1 : Gain  Gain=latsys.a  Multiplication=Matrix(K*u)
  B : Gain  Gain=longsys.b  Multiplication=Matrix(K*u)
  B1 : Gain  Gain=latsys.b  Multiplication=Matrix(K*u)
  Constant : Constant  Value=0
  Integrator : Integrator
  Integrator1 : Integrator
  K_lat : Gain  Gain=-K_lat  Multiplication=Matrix(K*u)
  K_long : Gain  Gain=-K_long  Multiplication=Matrix(K*u)
  Ke_long : Gain  Gain=Kobsvlong  Multiplication=Matrix(K*u)
  Ke_long1 : Gain  Gain=Kobsvlat  Multiplication=Matrix(K*u)
  Mux : Mux  Inputs=2
  Scope3 : Scope
  Selector1 : Selector  InputPortWidth=9  IndexOptions=Index vector (dialog)  Indices=[5:9]  OutputSizes=1
  Selector2 : Selector  InputPortWidth=4  IndexOptions=Index vector (dialog)  Indices=[3:4]  OutputSizes=1
  Selector3 : Selector  InputPortWidth=9  IndexOptions=Index vector (dialog)  Indices=[1:4]  OutputSizes=1
  Selector4 : Selector  InputPortWidth=4  IndexOptions=Index vector (dialog)  Indices=[1]  OutputSizes=1
  Sum : Sum  Inputs=-+|
  Sum{1..4} (4 alike) : Sum  Inputs=|++
  Sum5 : Sum  Inputs=-+|
  Sum6 : Sum  Inputs=|+-
  U1 : InportShadow  Port=2  PortDimensions=[4,1]
  c : Gain  Gain=long.c  Multiplication=Matrix(K*u)
  c1 : Gain  Gain=lat.c  Multiplication=Matrix(K*u)
  lat.c : Gain  Gain=lat.c  Multiplication=Matrix(K*u)
  long.c : Gain  Gain=long.c  Multiplication=Matrix(K*u)
  Longitudinal Control : Outport
  Lateral-Directional Control : Outport  Port=2
  wires:
  Constant/1 -> Mux/2
  K_long/1 -> Mux/1  "u_long"
  Mux/1 -> Longitudinal Control/1
  Selector2/1 -> B1/1
  Selector4/1 -> B/1
  U1/1 -> Selector2/1
  U/1 -> Selector4/1
  Sum6/1 -> Scope3/1
  c1/1 -> Sum5/1
  B1/1 -> Sum4/2
  A1/1 -> Sum3/2
  Sum3/1 -> Integrator1/1
  Sum4/1 -> Sum3/1
  Ke_long1/1 -> Sum4/1
  Sum5/1 -> Ke_long1/1
  lat.c/1 -> Sum5/2  "y_lat"
  Integrator1/1 -> c1/1, A1/1, K_lat/1
  c/1 -> Sum/1  "y^"
  long.c/1 -> Sum/2  "y_long"
  A/1 -> Sum2/2
  Integrator/1 -> Sum6/2, c/1, K_long/1, A/1
  Sum2/1 -> Integrator/1
  Sum1/1 -> Sum2/1
  B/1 -> Sum1/2
  Ke_long/1 -> Sum1/1
  Sum/1 -> Ke_long/1
  States/1 -> Selector3/1, Selector1/1
  Selector3/1 -> Sum6/1, long.c/1  "Longitudinal"
  Selector1/1 -> lat.c/1  "Lateral-Directional"
  K_lat/1 -> Lateral-Directional Control/1

== system AFDNFSmodelSPA/OnBoardComputer/Control System/Unfinished Controllers (State-Feedback)/Reduced Order Observer Servo ==
  States : Inport  PortDimensions=[9,1]
  A : Gain  Gain=longsys.a  Multiplication=Matrix(K*u)
  A1 : Gain  Gain=latsys.a  Multiplication=Matrix(K*u)
  B : Gain  Gain=longsys.b  Multiplication=Matrix(K*u)
  B1 : Gain  Gain=latsys.b  Multiplication=Matrix(K*u)
  Integrator : Integrator
  Integrator1 : Integrator
  K_lat : Gain  Gain=-K_lat  Multiplication=Matrix(K*u)
  K_long : Gain  Gain=-K_long  Multiplication=Matrix(K*u)
  Ke_long : Gain  Gain=Kobsvlong  Multiplication=Matrix(K*u)
  Ke_long1 : Gain  Gain=Kobsvlat  Multiplication=Matrix(K*u)
  Selector1 : Selector  InputPortWidth=9  IndexOptions=Index vector (dialog)  Indices=[5:9]  OutputSizes=1
  Selector3 : Selector  InputPortWidth=9  IndexOptions=Index vector (dialog)  Indices=[1:4]  OutputSizes=1
  Sum : Sum  Inputs=-+|
  Sum1 : Sum  Inputs=|++
  Sum2 : Sum  Inputs=|+-
  Sum3 : Sum  Inputs=|+-
  Sum4 : Sum  Inputs=|++
  Sum5 : Sum  Inputs=-+|
  c : Gain  Gain=long.c  Multiplication=Matrix(K*u)
  c1 : Gain  Gain=lat.c  Multiplication=Matrix(K*u)
  lat.c : Gain  Gain=lat.c  Multiplication=Matrix(K*u)
  long.c : Gain  Gain=long.c  Multiplication=Matrix(K*u)
  Longitudinal Control : Outport
  Lateral-Directional Control : Outport  Port=2
  wires:
  K_lat/1 -> Lateral-Directional Control/1, B1/1
  K_long/1 -> Longitudinal Control/1, B/1  "u_long"
  Selector1/1 -> lat.c/1  "Lateral-Directional"
  Selector3/1 -> long.c/1  "Longitudinal"
  States/1 -> Selector1/1, Selector3/1
  Sum/1 -> Ke_long/1
  Ke_long/1 -> Sum1/1
  B/1 -> Sum1/2
  Sum1/1 -> Sum2/1
  Sum2/1 -> Integrator/1
  Integrator/1 -> A/1, K_long/1, c/1
  A/1 -> Sum2/2
  long.c/1 -> Sum/2  "y_long"
  c/1 -> Sum/1
  Integrator1/1 -> K_lat/1, A1/1, c1/1
  lat.c/1 -> Sum5/2  "y_lat"
  Sum5/1 -> Ke_long1/1
  Ke_long1/1 -> Sum4/1
  Sum4/1 -> Sum3/1
  Sum3/1 -> Integrator1/1
  A1/1 -> Sum3/2
  B1/1 -> Sum4/2
  c1/1 -> Sum5/1

== system AFDNFSmodelSPA/Nonlinear Flight Simulator/6DoF Nonlinear Flight Equations of Motion (Rigid Body)/AngularAcceleration(Omegadot)/Cross Product/Subsystem2 ==
  A : Inport
  B : Inport  Port=2
  Demux : Demux  Outputs=3
  Demux1 : Demux  Outputs=3
  Mux : Mux  Inputs=3
  i x j : Product  SaturateOnIntegerOverflow=on  InputSameDT=on  OutDataTypeStr=Inherit: Same as first input
  j x k : Product  SaturateOnIntegerOverflow=on  InputSameDT=on  OutDataTypeStr=Inherit: Same as first input
  k x i : Product  SaturateOnIntegerOverflow=on  InputSameDT=on  OutDataTypeStr=Inherit: Same as first input
  Out1 : Outport
  wires:
  Demux1/3 -> j x k/2
  Demux/2 -> j x k/1
  Demux/3 -> k x i/1
  Demux1/1 -> k x i/2
  Demux1/2 -> i x j/2
  Demux/1 -> i x j/1
  i x j/1 -> Mux/3
  k x i/1 -> Mux/2
  j x k/1 -> Mux/1
  B/1 -> Demux1/1
  A/1 -> Demux/1
  Mux/1 -> Out1/1

== system AFDNFSmodelSPA/Nonlinear Flight Simulator/6DoF Nonlinear Flight Equations of Motion (Rigid Body)/AngularAcceleration(Omegadot)/Cross Product/Subsystem3 ==
  A : Inport
  B : Inport  Port=2
  Demux : Demux  Outputs=3
  Demux1 : Demux  Outputs=3
  Mux : Mux  Inputs=3
  i x k : Product  SaturateOnIntegerOverflow=on  InputSameDT=on  OutDataTypeStr=Inherit: Same as first input
  j x i : Product  SaturateOnIntegerOverflow=on  InputSameDT=on  OutDataTypeStr=Inherit: Same as first input
  k x j : Product  SaturateOnIntegerOverflow=on  InputSameDT=on  OutDataTypeStr=Inherit: Same as first input
  Out2 : Outport
  wires:
  j x i/1 -> Mux/3
  i x k/1 -> Mux/2
  k x j/1 -> Mux/1
  Mux/1 -> Out2/1
  Demux1/1 -> j x i/2
  Demux/2 -> j x i/1
  Demux1/3 -> i x k/2
  Demux/1 -> i x k/1
  Demux1/2 -> k x j/2
  Demux/3 -> k x j/1
  B/1 -> Demux1/1
  A/1 -> Demux/1

== system AFDNFSmodelSPA/Nonlinear Flight Simulator/6DoF Nonlinear Flight Equations of Motion (Rigid Body)/Linear Acceleration(Vdot)/Cross Product/Subsystem2 ==
  A : Inport
  B : Inport  Port=2
  Demux : Demux  Outputs=3
  Demux1 : Demux  Outputs=3
  Mux : Mux  Inputs=3
  i x j : Product  SaturateOnIntegerOverflow=on  InputSameDT=on  OutDataTypeStr=Inherit: Same as first input
  j x k : Product  SaturateOnIntegerOverflow=on  InputSameDT=on  OutDataTypeStr=Inherit: Same as first input
  k x i : Product  SaturateOnIntegerOverflow=on  InputSameDT=on  OutDataTypeStr=Inherit: Same as first input
  Out1 : Outport
  wires:
  Demux1/3 -> j x k/2
  Demux/2 -> j x k/1
  Demux/3 -> k x i/1
  Demux1/1 -> k x i/2
  Demux1/2 -> i x j/2
  Demux/1 -> i x j/1
  i x j/1 -> Mux/3
  k x i/1 -> Mux/2
  j x k/1 -> Mux/1
  B/1 -> Demux1/1
  A/1 -> Demux/1
  Mux/1 -> Out1/1

== system AFDNFSmodelSPA/Nonlinear Flight Simulator/6DoF Nonlinear Flight Equations of Motion (Rigid Body)/Linear Acceleration(Vdot)/Cross Product/Subsystem3 ==
  A : Inport
  B : Inport  Port=2
  Demux : Demux  Outputs=3
  Demux1 : Demux  Outputs=3
  Mux : Mux  Inputs=3
  i x k : Product  SaturateOnIntegerOverflow=on  InputSameDT=on  OutDataTypeStr=Inherit: Same as first input
  j x i : Product  SaturateOnIntegerOverflow=on  InputSameDT=on  OutDataTypeStr=Inherit: Same as first input
  k x j : Product  SaturateOnIntegerOverflow=on  InputSameDT=on  OutDataTypeStr=Inherit: Same as first input
  Out2 : Outport
  wires:
  j x i/1 -> Mux/3
  i x k/1 -> Mux/2
  k x j/1 -> Mux/1
  Mux/1 -> Out2/1
  Demux1/1 -> j x i/2
  Demux/2 -> j x i/1
  Demux1/3 -> i x k/2
  Demux/1 -> i x k/1
  Demux1/2 -> k x j/2
  Demux/3 -> k x j/1
  B/1 -> Demux1/1
  A/1 -> Demux/1
